simulink model "FullSystemSimGoed"  (R2020a)
settings: Solver=VariableStepAuto  StartTime=0.0  StopTime=T_sim  RelTol=1e-3
values from neighbouring files (symbols this model uses):
  a_friction = 0    [FullSystem.m]
  b_friction = 1.19    [FullSystem.m]
  C_T_matrix = ex2(2:12,2:12)'    [FullSystem.m]
  d_turbine = 0.15    [FullSystem.m]
  J_wind = 5.245e-6 * 1000    (= 0.005245)    [FullSystem.m]
  K_t = 0.023    [FullSystem.m]    (also in WindTurbine.m = 82.8991502528)
  K_v = 0.023 * pi / 30    (= 0.00240855436775)    [FullSystem.m]    (also in WindTurbine.m = 115.191730632)
  lambda_data_x = ex3(3, :)'    [FullSystem.m]
  lambda_opt = 2.8    [FullSystem.m]
  omega_0 = 1000    [FullSystem.m]    (also in SystemControl_script.m = 100:)
  P_max_EL = 3    [FullSystem.m]
  P_max_FC = 1    [FullSystem.m]
  P_max_LED = 12*0.16*4    (= 7.68)    [FullSystem.m]
  P_max_SP = 0.5    [FullSystem.m]
  P_max_WT = 0.2    [FullSystem.m]
  R_LED_max = 75/4    (= 18.75)    [FullSystem.m]
  r_LED_x = ex1(4, :)'    [FullSystem.m]
  r_PS_x = ex1(5,:)'    [FullSystem.m]
  r_SP_x = ex1(3, :)'    [FullSystem.m]
  r_wind_data_x = ex3(1, :)'    [FullSystem.m]
  r_WT_x = ex1(2, :)'    [FullSystem.m]
  rho_air = 1.225    [FullSystem.m]
  step_size = T_sim/n    (= 0.01)    [FullSystem.m]
  t_sample = pwm_timer/10    (= 0.01)    [FullSystem.m]
  T_sim = 10    [FullSystem.m]    (also in SystemControl_script.m; model_1.m = 24)
  V_w_data_x = ex3(2,:)'    [FullSystem.m]
undefined symbols (not defined in the file or in its folder): DiscIntNeverNeededParam
libraries: fl_lib x66, nesl_utility x55, ee_lib x12, eePwmGenerator x4, simulink x2
(part 1 of 2)
settings Model: Creator=thequ  LastModifiedBy=thequ
settings SolverCC: AlgebraicLoopSolver=LineSearch
settings DebuggingCC: ArithmeticOperatorsInVariantConditions=warning
settings SFSimCC: CustomCodeUndefinedFunction=UseInterfaceOnly

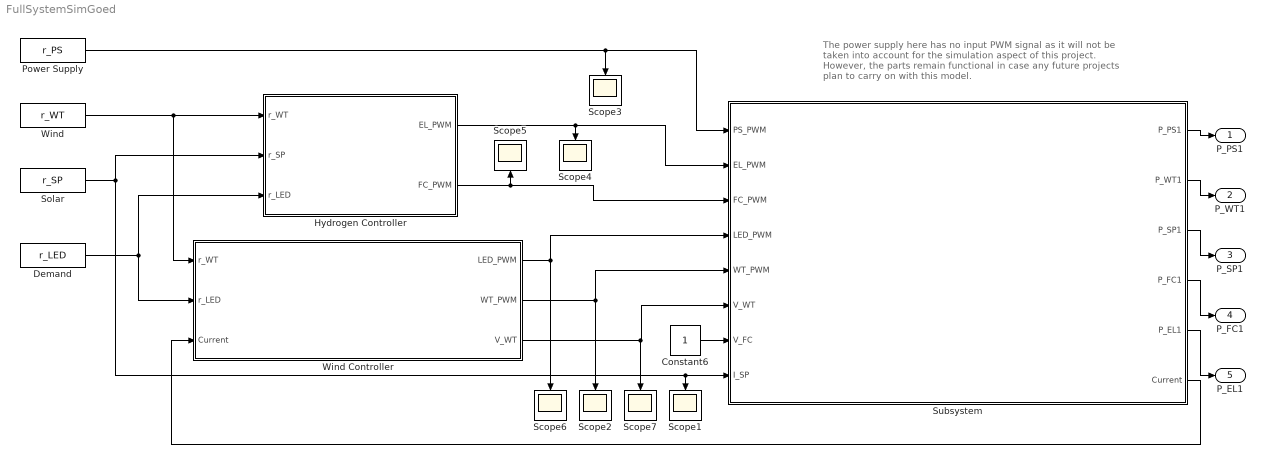
== system FullSystemSimGoed ==
  note: The power supply here has no input PWM signal as it will not
      | be taken into account for the simulation aspect of this project.
      | However, the parts remain functional in case any future
      | projects plan to carry on with this model.
  Constant6 : Constant
  Demand : FromWorkspace  VariableName=r_LED  SampleTime=T_sim/length(r_LED_x)  Interpolate=off  OutputAfterFinalValue=Holding final value
  Hydrogen Controller : Subsystem
  Power Supply : FromWorkspace  VariableName=r_PS  SampleTime=T_sim/length(r_PS_x)  Interpolate=off  OutputAfterFinalValue=Holding final value
  Scope{1..7} (7 alike) : Scope
  Solar : FromWorkspace  VariableName=r_SP  SampleTime=T_sim/length(r_SP_x)  Interpolate=off  OutputAfterFinalValue=Holding final value
  Subsystem : Subsystem
  Wind : FromWorkspace  VariableName=r_WT  SampleTime=T_sim/length(r_WT_x)  Interpolate=off  OutputAfterFinalValue=Holding final value
  Wind Controller : Subsystem
  P_PS1 : Outport
  P_WT1 : Outport  Port=2
  P_SP1 : Outport  Port=3
  P_FC1 : Outport  Port=4
  P_EL1 : Outport  Port=5
  wires:
  Subsystem/1(P_PS1) -> P_PS1/1
  Subsystem/2(P_WT1) -> P_WT1/1
  Subsystem/3(P_SP1) -> P_SP1/1
  Subsystem/4(P_FC1) -> P_FC1/1
  Subsystem/5(P_EL1) -> P_EL1/1
  Demand/1 -> Hydrogen Controller/3(r_LED), Wind Controller/2(r_LED)
  Constant6/1 -> Subsystem/7(V_FC)
  Wind/1 -> Wind Controller/1(r_WT), Hydrogen Controller/1(r_WT)
  Solar/1 -> Hydrogen Controller/2(r_SP), Subsystem/8(I_SP), Scope1/1
  Wind Controller/2(WT_PWM) -> Scope2/1, Subsystem/5(WT_PWM)
  Power Supply/1 -> Subsystem/1(PS_PWM), Scope3/1
  Hydrogen Controller/1(EL_PWM) -> Subsystem/2(EL_PWM), Scope4/1
  Hydrogen Controller/2(FC_PWM) -> Subsystem/3(FC_PWM), Scope5/1
  Wind Controller/1(LED_PWM) -> Scope6/1, Subsystem/4(LED_PWM)
  Wind Controller/3(V_WT) -> Scope7/1, Subsystem/6(V_WT)
  Subsystem/6(Current) -> Wind Controller/3(Current)

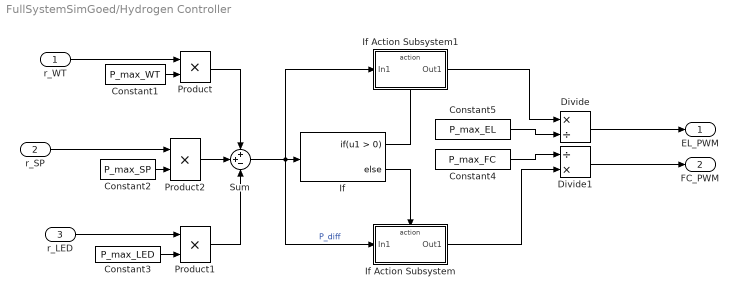
== system FullSystemSimGoed/Hydrogen Controller ==
  r_WT : Inport
  r_SP : Inport  Port=2
  r_LED : Inport  Port=3
  Constant1 : Constant  Value=P_max_WT
  Constant2 : Constant  Value=P_max_SP
  Constant3 : Constant  Value=P_max_LED
  Constant4 : Constant  Value=P_max_FC
  Constant5 : Constant  Value=P_max_EL
  Divide : Product  Inputs=*/
  Divide1 : Product  Inputs=/*
  If : If
  If Action Subsystem : Subsystem  TreatAsAtomicUnit=on
  If Action Subsystem1 : Subsystem  TreatAsAtomicUnit=on
  Product : Product
  Product1 : Product
  Product2 : Product
  Sum : Sum  Inputs=++-
  EL_PWM : Outport
  FC_PWM : Outport  Port=2
  wires:
  Divide1/1 -> FC_PWM/1
  Product/1 -> Sum/1
  Divide/1 -> EL_PWM/1
  r_WT/1 -> Product/1
  If Action Subsystem/1(Out1) -> Divide1/2
  Constant5/1 -> Divide/2
  If/2 -> If Action Subsystem/Action
  Product1/1 -> Sum/3
  Sum/1 -> If Action Subsystem1/1(In1), If Action Subsystem/1(In1), If/1  "P_diff"
  Constant1/1 -> Product/2
  Constant4/1 -> Divide1/1
  If/1 -> If Action Subsystem1/Action
  If Action Subsystem1/1(Out1) -> Divide/1
  Constant3/1 -> Product1/2
  Constant2/1 -> Product2/2
  Product2/1 -> Sum/2
  r_LED/1 -> Product1/1
  r_SP/1 -> Product2/1

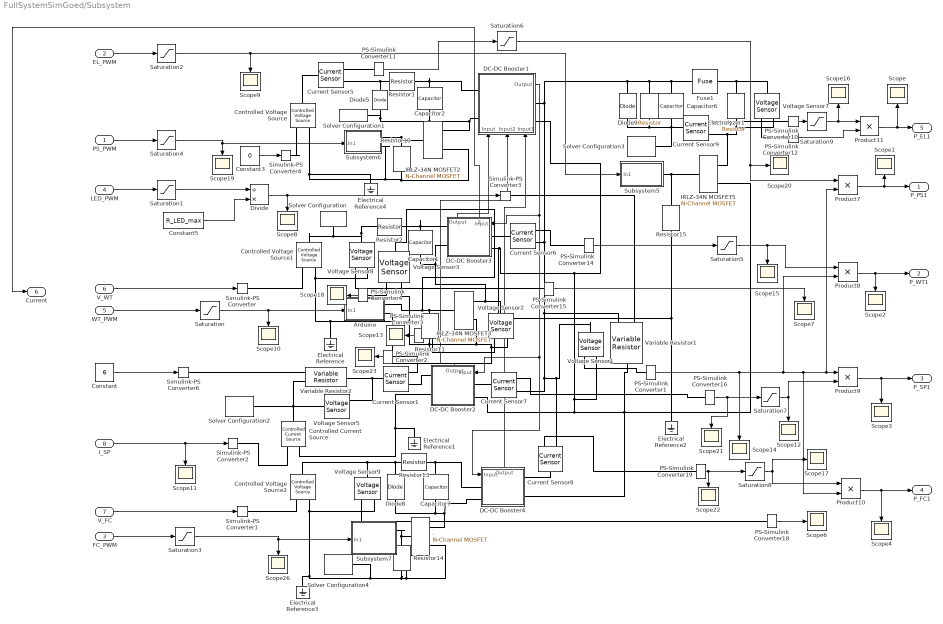
== system FullSystemSimGoed/Subsystem ==
  PS_PWM : Inport
  EL_PWM : Inport  Port=2
  FC_PWM : Inport  Port=3
  LED_PWM : Inport  Port=4
  WT_PWM : Inport  Port=5
  V_WT : Inport  Port=6
  V_FC : Inport  Port=7
  I_SP : Inport  Port=8
  " " : fl_lib/Electrical/Electrical Elements/Resistor  R=16 Ohm  i_specify=off  i_priority=None  i=0 A  i_nominal_specify=off  i_nominal_unit=A  i_nominal_value=1  v_specify=off  v_priority=None  v=0 V  v_nominal_specify=off  v_nominal_unit=V  v_nominal_value=1
  . : ee_lib/Semiconductors & Converters/N-Channel MOSFET  paramTerminal=ee.enum.mosfet.numberOfTerminals.three  parameterization=1  prmDatasheet=1  prmEquCoeff=1  Beta=5.0 A/V^2  Rds=0.046 Ohm  Id=30 A  Vgs=5 V  Vth=1.5 V  Vth0=1.7 V  lam=0 1/V  gamma_vth=0.5 V^0.50000  phib=0.5 V  Vth1=1.9071 V  Vbs1=-1 V  Vth2=2.066 V  Vbs2=-2 V  Tmeas=25 degC  RS=0.0001 Ohm  RD=0.01 Ohm  RB=0.001 Ohm  C_param=1  C_GS=270 pF  C_GD=80 pF  C_DS=0 pF  C_iss=350 pF  C_rss=80 pF  C_oss=0 pF  charge_linearity_param=1  C_OX=200 pF  V_C_OX=-0.5 V  C_iss_vec=[720, 700, 590, 470, 390, 310] pF  C_rss_vec=[450, 400, 300, 190, 95, 55] pF  C_oss_vec=[900, 810, 690, 420, 270, 170] pF  C_GS_vec=[270, 300, 290, 280, 295, 255] pF  C_GD_vec=[450, 400, 300, 190, 95, 55] pF  C_DS_vec=[450, 410, 390, 230, 175, 115] pF  C_Vds_vec=[.1, .3, 1, 3, 10, 30] V  V_GS_for_cap_data=0 V  charge_linearity_param_vgb=ee.enum.mosfet.cgbLinearity.instantly  IsDiode=0 A  Vbi=0.6 V  n=1  Cj0Diode=0 pF  TT=50e-9 s  dVth_dT=-6 mV/K  dVth0_dT=-6 mV/K  Rds_T2=0.037 Ohm  Tmeas2=125 degC  BEXDatasheet=-1.5  BEXEquCoeff=-1.5  etaisDatasheet=3  etaisEquCoeff=3  TdeviceDatasheet=25 degC  TdeviceEquCoeff=25 degC  thermal_network_parameterization=ee.enum.thermalNetworkTopology.cauer  Rth=[0, 10] K/W  Rth_Foster=[4, 6] K/W  thermal_mass_parameterization=ee.enum.thermalNetwork.timeconstant  thermal_mass=[0, 1] J/K  thermal_mass_Foster=[1.5, 3] J/K  thermal_time_constant=[0, 10] s  thermal_time_constant_Foster=[6, 18] s  thermal_mass_initial_temperatures=[25, 25] degC  betaref=18 A/V^2  Vfbref=-1.1 V  gamma=3.5 V^0.50000  phib2ref=1 V  thesatref=0.4 1/V  alpha=0  Vp=5e-2 V  thesrref=0 1/V  m=8  Tref=25 degC  Cox=1500 pF  Cgso=100 pF  Cgdo=14 pF  Rsref=2e-3 Ohm  Rdref=0.17 Ohm  Rgref=8.4 Ohm  Rbref=2e-3 Ohm  Isref=5.2e-13 A  Cj0=480 pF  Tprm=1  etabet=1.3  Stvfb=5e-4 V/K  Stphib=-8.5e-4 V/K  etasat=1.04  etasr=0.65  etar=0.95  etais=3  Tsim=25 degC  T0=[25, 25] degC
  Arduino : Subsystem
  Capacitor1 : fl_lib/Electrical/Electrical Elements/Capacitor  c=1000 uF  r=0.02 Ohm  g=0 1/Ohm  i_specify=off  i_priority=None  i=0 A  i_nominal_specify=off  i_nominal_unit=A  i_nominal_value=1  v_specify=off  v_priority=None  v=0 V  v_nominal_specify=off  v_nominal_unit=V  v_nominal_value=1  vc_specify=off  vc_priority=High  vc=0 V  vc_nominal_specify=off  vc_nominal_unit=V  vc_nominal_value=1
  Capacitor2 : fl_lib/Electrical/Electrical Elements/Capacitor  c=1000 uF  r=0.02 Ohm  g=0 1/Ohm  i_specify=off  i_priority=None  i=0 A  i_nominal_specify=off  i_nominal_unit=A  i_nominal_value=1  v_specify=off  v_priority=None  v=0 V  v_nominal_specify=off  v_nominal_unit=V  v_nominal_value=1  vc_specify=off  vc_priority=High  vc=0 V  vc_nominal_specify=off  vc_nominal_unit=V  vc_nominal_value=1
  Capacitor6 : fl_lib/Electrical/Electrical Elements/Capacitor  c=1000 uF  r=0.20 Ohm  g=0 1/Ohm  i_specify=off  i_priority=None  i=0 A  i_nominal_specify=off  i_nominal_unit=A  i_nominal_value=1  v_specify=off  v_priority=None  v=0 V  v_nominal_specify=off  v_nominal_unit=V  v_nominal_value=1  vc_specify=off  vc_priority=High  vc=0 V  vc_nominal_specify=off  vc_nominal_unit=V  vc_nominal_value=1
  Capacitor7 : fl_lib/Electrical/Electrical Elements/Capacitor  c=1000 uF  r=0.02 Ohm  g=0 1/Ohm  i_specify=off  i_priority=None  i=0 A  i_nominal_specify=off  i_nominal_unit=A  i_nominal_value=1  v_specify=off  v_priority=None  v=0 V  v_nominal_specify=off  v_nominal_unit=V  v_nominal_value=1  vc_specify=off  vc_priority=High  vc=0 V  vc_nominal_specify=off  vc_nominal_unit=V  vc_nominal_value=1
  Constant : Constant  Value=6
  Constant3 : Constant  Value=0
  Constant5 : Constant  Value=R_LED_max
  Controlled Current Source : fl_lib/Electrical/Electrical Sources/Controlled Current Source
  Controlled Voltage Source : fl_lib/Electrical/Electrical Sources/Controlled Voltage Source
  Controlled Voltage Source1 : fl_lib/Electrical/Electrical Sources/Controlled Voltage Source
  Controlled Voltage Source2 : fl_lib/Electrical/Electrical Sources/Controlled Voltage Source
  Current Sensor{1,5..9} (6 alike) : fl_lib/Electrical/Electrical Sensors/Current Sensor
  DC-DC Booster1 : Subsystem
      settings: PortSchema="{\"entries\":[{\"content\":{\"sides\":[{\"content\":{\"connectorIds\":[\"LConn1\",\"LConn2\"]},\"type\":\"ConnectorPlacement.EquallySpacedRectSide\",\"uuid\":\"3f87025d-e72c-4f7c-9c78-5492fcc5bb7b\"},{\"content\":{\"connectorIds\":[\"Out1\",\"RConn1\",\"RConn2\"],\"side\":\"RIGHT\"},\"type\":\"ConnectorPlacement.EquallySpacedRectSide\",\"uuid\":\"8496db32-d1b8-4ca7-babe-2510a055e486\"},{\"content\":{\"connectorIds\":[],\"side\":\"TOP\"},\"type\":\"ConnectorPlacement.EquallySpacedRectSide\",\"uuid\":\"d85b2c98-f560-4129-a6ac-6fa684551bcf\"},{\"content\":{\"connectorIds\":[\"In1\",\"In2\",\"In3\"],\"side\":\"BOTTOM\"},\"type\":\"ConnectorPlacement.EquallySpacedRectSide\",\"uuid\":\"fe0eaf9c-8c75-4de4-84e6-0314a1617f55\"}]},\"type\":\"ConnectorPlacement.EquallySpacedConnector\",\"uuid\":\"a6ed506c-6875-4055-9614-7dad2b572790\"}],\"packageUris\":[\"http://schema.mathworks.com/mf0/Connector/19700101\"],\"version\":\"1.0\"}"
  DC-DC Booster2 : Subsystem
      settings: PortSchema="{\"entries\":[{\"content\":{\"sides\":[{\"content\":{\"connectorIds\":[\"LConn1\",\"LConn2\"]},\"type\":\"ConnectorPlacement.EquallySpacedRectSide\",\"uuid\":\"e779e15f-05fe-47ae-aa08-5379ba170b98\"},{\"content\":{\"connectorIds\":[\"In1\",\"RConn1\",\"RConn2\"],\"side\":\"RIGHT\"},\"type\":\"ConnectorPlacement.EquallySpacedRectSide\",\"uuid\":\"c806a98b-8847-4c98-ba30-df3a6a47e20e\"},{\"content\":{\"connectorIds\":[\"Out1\"],\"side\":\"TOP\"},\"type\":\"ConnectorPlacement.EquallySpacedRectSide\",\"uuid\":\"f525c8fa-41c3-4ddc-a882-4dcfcc470e8d\"}]},\"type\":\"ConnectorPlacement.EquallySpacedConnector\",\"uuid\":\"8e1dab04-976c-405f-8e86-df668b770438\"}],\"packageUris\":[\"http://schema.mathworks.com/mf0/Connector/19700101\"],\"version\":\"1.0\"}"
  DC-DC Booster3 : Subsystem
      settings: PortSchema="{\"entries\":[{\"content\":{\"sides\":[{\"content\":{\"connectorIds\":[\"LConn1\",\"LConn2\"]},\"type\":\"ConnectorPlacement.EquallySpacedRectSide\",\"uuid\":\"e779e15f-05fe-47ae-aa08-5379ba170b98\"},{\"content\":{\"connectorIds\":[\"In1\",\"RConn1\",\"RConn2\"],\"side\":\"RIGHT\"},\"type\":\"ConnectorPlacement.EquallySpacedRectSide\",\"uuid\":\"c806a98b-8847-4c98-ba30-df3a6a47e20e\"},{\"content\":{\"connectorIds\":[\"Out1\",\"Out2\"],\"side\":\"TOP\"},\"type\":\"ConnectorPlacement.EquallySpacedRectSide\",\"uuid\":\"f525c8fa-41c3-4ddc-a882-4dcfcc470e8d\"}]},\"type\":\"ConnectorPlacement.EquallySpacedConnector\",\"uuid\":\"8e1dab04-976c-405f-8e86-df668b770438\"}],\"packageUris\":[\"http://schema.mathworks.com/mf0/Connector/19700101\"],\"version\":\"1.0\"}"
  DC-DC Booster4 : Subsystem
      settings: PortSchema="{\"entries\":[{\"content\":{\"sides\":[{\"content\":{\"connectorIds\":[\"In1\",\"LConn1\",\"LConn2\"]},\"type\":\"ConnectorPlacement.EquallySpacedRectSide\",\"uuid\":\"53e27ef1-b6e4-4838-a313-2833a9f48f28\"},{\"content\":{\"connectorIds\":[\"RConn1\",\"RConn2\"],\"side\":\"RIGHT\"},\"type\":\"ConnectorPlacement.EquallySpacedRectSide\",\"uuid\":\"d6eb4206-926e-4a9e-8f3b-898e00b2f09a\"},{\"content\":{\"connectorIds\":[\"Out1\"],\"side\":\"TOP\"},\"type\":\"ConnectorPlacement.EquallySpacedRectSide\",\"uuid\":\"2a6192b7-9850-4397-b133-a2a3e44eb736\"}]},\"type\":\"ConnectorPlacement.EquallySpacedConnector\",\"uuid\":\"90d1bf23-e581-4b0f-8608-623e9f776cda\"}],\"packageUris\":[\"http://schema.mathworks.com/mf0/Connector/19700101\"],\"version\":\"1.0\"}"
  Diode5 : ee_lib/Semiconductors & Converters/Diode  ModelType=ee.enum.diode.modelType.pwl  Vf=0.6 V  Ron=0.3 Ohm  Goff=1e-8 S  prmExp=ee.enum.diode.expParam.useTwo  I12=[.0137, .545] A  V12=[.6, .7] V  IS=1e-12 A  ec=1  I1=0.0137 A  V1=0.6 V  RS=0 Ohm  Tmeas=25 degC  N_series=1  N_parallel=1  Rz=0.3 Ohm  BV=inf V  C_param=ee.enum.diode.capParam.fixed  CJ=5 pF  CJ0=5 pF  VJ=1 V  Mgrad=0.5  Vvec=[.1, 10, 100] V  Cvec=[3.5, 1, .4] pF  FC=0.5  Q_param=ee.enum.diode.recoveryParam.off  iRM=-7.15 A  iF=4 A  didt=-750 A/us  trr_factor=3  trr=115 ns  Qrr=1500 s*uA  TT=50 ns  tau=100 ns  T_param=ee.enum.diode.temperatureParam.off  IS_T2=1.25e-7 A  I1_T2=0.245 A  V1_T2=0.5 V  Tmeas2=125 degC  EG_param=ee.enum.diode.egapParam.material_si  EG=1.11 eV  XTI_param=ee.enum.diode.xtiParam.pn  XTI=3  dBVdT=0 V/K  Tdevice=25 degC  i_specify=off  i_priority=None  i=0 A  i_nominal_specify=off  i_nominal_unit=A  i_nominal_value=1  v_specify=off  v_priority=None  v=0 V  v_nominal_specify=off  v_nominal_unit=V  v_nominal_value=1  i_capacitor_specify=off  i_capacitor_priority=None  i_capacitor=0 A  i_capacitor_nominal_specify=off  i_capacitor_nominal_unit=A  i_capacitor_nominal_value=1  v_capacitor_specify=off  v_capacitor_priority=None  v_capacitor=0 V  v_capacitor_nominal_specify=off  v_capacitor_nominal_unit=V  v_capacitor_nominal_value=1  power_dissipated_specify=off  power_dissipated_priority=None  power_dissipated=0 W  power_dissipated_nominal_specify=off  power_dissipated_nominal_unit=W  power_dissipated_nominal_value=1  thermal_network_parameterization=ee.enum.thermalNetworkTopology.cauer  Rth=[0, 10] K/W  Rth_Foster=[4, 6] K/W  thermal_mass_parameterization=ee.enum.thermalNetwork.timeconstant  thermal_mass=[0, 1] J/K  thermal_mass_Foster=[1.5, 3] J/K  thermal_time_constant=[0, 10] s  thermal_time_constant_Foster=[6, 18] s  thermal_mass_initial_temperatures=[25, 25] degC
  Diode8 : ee_lib/Semiconductors & Converters/Diode  ModelType=ee.enum.diode.modelType.pwl  Vf=0.85 V  Ron=0.05 Ohm  Goff=1e-8 S  prmExp=ee.enum.diode.expParam.useTwo  I12=[.0137, .545] A  V12=[.6, .7] V  IS=1e-12 A  ec=1  I1=0.0137 A  V1=0.6 V  RS=0 Ohm  Tmeas=25 degC  N_series=1  N_parallel=1  Rz=0.3 Ohm  BV=inf V  C_param=ee.enum.diode.capParam.fixed  CJ=5 pF  CJ0=5 pF  VJ=1 V  Mgrad=0.5  Vvec=[.1, 10, 100] V  Cvec=[3.5, 1, .4] pF  FC=0.5  Q_param=ee.enum.diode.recoveryParam.off  iRM=-7.15 A  iF=4 A  didt=-750 A/us  trr_factor=3  trr=115 ns  Qrr=1500 s*uA  TT=50 ns  tau=100 ns  T_param=ee.enum.diode.temperatureParam.off  IS_T2=1.25e-7 A  I1_T2=0.245 A  V1_T2=0.5 V  Tmeas2=125 degC  EG_param=ee.enum.diode.egapParam.material_si  EG=1.11 eV  XTI_param=ee.enum.diode.xtiParam.pn  XTI=3  dBVdT=0 V/K  Tdevice=25 degC  i_specify=off  i_priority=None  i=0 A  i_nominal_specify=off  i_nominal_unit=A  i_nominal_value=1  v_specify=off  v_priority=None  v=0 V  v_nominal_specify=off  v_nominal_unit=V  v_nominal_value=1  i_capacitor_specify=off  i_capacitor_priority=None  i_capacitor=0 A  i_capacitor_nominal_specify=off  i_capacitor_nominal_unit=A  i_capacitor_nominal_value=1  v_capacitor_specify=off  v_capacitor_priority=None  v_capacitor=0 V  v_capacitor_nominal_specify=off  v_capacitor_nominal_unit=V  v_capacitor_nominal_value=1  power_dissipated_specify=off  power_dissipated_priority=None  power_dissipated=0 W  power_dissipated_nominal_specify=off  power_dissipated_nominal_unit=W  power_dissipated_nominal_value=1  thermal_network_parameterization=ee.enum.thermalNetworkTopology.cauer  Rth=[0, 10] K/W  Rth_Foster=[4, 6] K/W  thermal_mass_parameterization=ee.enum.thermalNetwork.timeconstant  thermal_mass=[0, 1] J/K  thermal_mass_Foster=[1.5, 3] J/K  thermal_time_constant=[0, 10] s  thermal_time_constant_Foster=[6, 18] s  thermal_mass_initial_temperatures=[25, 25] degC
  Diode9 : ee_lib/Semiconductors & Converters/Diode  ModelType=ee.enum.diode.modelType.pwl  Vf=0.7 V  Ron=0.3 Ohm  Goff=1e-8 S  prmExp=ee.enum.diode.expParam.useTwo  I12=[.0137, .545] A  V12=[.6, .7] V  IS=1e-12 A  ec=1  I1=0.0137 A  V1=0.6 V  RS=0 Ohm  Tmeas=25 degC  N_series=1  N_parallel=1  Rz=0.3 Ohm  BV=inf V  C_param=ee.enum.diode.capParam.fixed  CJ=5 pF  CJ0=5 pF  VJ=1 V  Mgrad=0.5  Vvec=[.1, 10, 100] V  Cvec=[3.5, 1, .4] pF  FC=0.5  Q_param=ee.enum.diode.recoveryParam.off  iRM=-7.15 A  iF=4 A  didt=-750 A/us  trr_factor=3  trr=115 ns  Qrr=1500 s*uA  TT=50 ns  tau=100 ns  T_param=ee.enum.diode.temperatureParam.off  IS_T2=1.25e-7 A  I1_T2=0.245 A  V1_T2=0.5 V  Tmeas2=125 degC  EG_param=ee.enum.diode.egapParam.material_si  EG=1.11 eV  XTI_param=ee.enum.diode.xtiParam.pn  XTI=3  dBVdT=0 V/K  Tdevice=25 degC  i_specify=off  i_priority=None  i=0 A  i_nominal_specify=off  i_nominal_unit=A  i_nominal_value=1  v_specify=off  v_priority=None  v=0 V  v_nominal_specify=off  v_nominal_unit=V  v_nominal_value=1  i_capacitor_specify=off  i_capacitor_priority=None  i_capacitor=0 A  i_capacitor_nominal_specify=off  i_capacitor_nominal_unit=A  i_capacitor_nominal_value=1  v_capacitor_specify=off  v_capacitor_priority=None  v_capacitor=0 V  v_capacitor_nominal_specify=off  v_capacitor_nominal_unit=V  v_capacitor_nominal_value=1  power_dissipated_specify=off  power_dissipated_priority=None  power_dissipated=0 W  power_dissipated_nominal_specify=off  power_dissipated_nominal_unit=W  power_dissipated_nominal_value=1  thermal_network_parameterization=ee.enum.thermalNetworkTopology.cauer  Rth=[0, 10] K/W  Rth_Foster=[4, 6] K/W  thermal_mass_parameterization=ee.enum.thermalNetwork.timeconstant  thermal_mass=[0, 1] J/K  thermal_mass_Foster=[1.5, 3] J/K  thermal_time_constant=[0, 10] s  thermal_time_constant_Foster=[6, 18] s  thermal_mass_initial_temperatures=[25, 25] degC
  Divide : Product  Inputs=/*
  Electrical Reference{,1..4} (5 alike) : fl_lib/Electrical/Electrical Elements/Electrical Reference
  Electrolyzer1 : fl_lib/Electrical/Electrical Elements/Resistor  R=4 Ohm  i_specify=off  i_priority=None  i=0 A  i_nominal_specify=off  i_nominal_unit=A  i_nominal_value=1  v_specify=off  v_priority=None  v=0 V  v_nominal_specify=off  v_nominal_unit=V  v_nominal_value=1
  Fuse1 : ee_lib/Switches & Breakers/Fuse  prm=1  I_rated=1.5 A  melt_margin=1  T_fuse=0 s  I2t=1 s*A^2  I_vec=[1.9, 2, 2.5, 30] A  t_vec=[10000, 1, .3, .001] s  R_closed=0.01 Ohm  G_open=1e-8 1/Ohm  exposemeasurement=ee.enum.exposemeasurement.hidden
      settings: SourceProductBaseCode=PS  InternalSimscapePortConfiguration="{\"Bottom\":[],\"Left\":[{\"id\":\"p\",\"label\":\"\",\"type\":\"foundation.electrical.electrical\"}],\"Right\":[{\"id\":\"n\",\"label\":\"\",\"type\":\"foundation.electrical.electrical\"}],\"Top\":[]}"
  IRLZ-34N MOSFET2 : ee_lib/Semiconductors & Converters/N-Channel MOSFET  paramTerminal=ee.enum.mosfet.numberOfTerminals.three  parameterization=1  prmDatasheet=1  prmEquCoeff=1  Beta=5.0 A/V^2  Rds=0.046 Ohm  Id=30 A  Vgs=5 V  Vth=1.5 V  Vth0=1.7 V  lam=0 1/V  gamma_vth=0.5 V^0.50000  phib=0.5 V  Vth1=1.9071 V  Vbs1=-1 V  Vth2=2.066 V  Vbs2=-2 V  Tmeas=25 degC  RS=0.0001 Ohm  RD=0.01 Ohm  RB=0.001 Ohm  C_param=1  C_GS=270 pF  C_GD=80 pF  C_DS=0 pF  C_iss=350 pF  C_rss=80 pF  C_oss=0 pF  charge_linearity_param=1  C_OX=200 pF  V_C_OX=-0.5 V  C_iss_vec=[720, 700, 590, 470, 390, 310] pF  C_rss_vec=[450, 400, 300, 190, 95, 55] pF  C_oss_vec=[900, 810, 690, 420, 270, 170] pF  C_GS_vec=[270, 300, 290, 280, 295, 255] pF  C_GD_vec=[450, 400, 300, 190, 95, 55] pF  C_DS_vec=[450, 410, 390, 230, 175, 115] pF  C_Vds_vec=[.1, .3, 1, 3, 10, 30] V  V_GS_for_cap_data=0 V  charge_linearity_param_vgb=ee.enum.mosfet.cgbLinearity.instantly  IsDiode=0 A  Vbi=0.6 V  n=1  Cj0Diode=0 pF  TT=50e-9 s  dVth_dT=-6 mV/K  dVth0_dT=-6 mV/K  Rds_T2=0.037 Ohm  Tmeas2=125 degC  BEXDatasheet=-1.5  BEXEquCoeff=-1.5  etaisDatasheet=3  etaisEquCoeff=3  TdeviceDatasheet=25 degC  TdeviceEquCoeff=25 degC  thermal_network_parameterization=ee.enum.thermalNetworkTopology.cauer  Rth=[0, 10] K/W  Rth_Foster=[4, 6] K/W  thermal_mass_parameterization=ee.enum.thermalNetwork.timeconstant  thermal_mass=[0, 1] J/K  thermal_mass_Foster=[1.5, 3] J/K  thermal_time_constant=[0, 10] s  thermal_time_constant_Foster=[6, 18] s  thermal_mass_initial_temperatures=[25, 25] degC  betaref=18 A/V^2  Vfbref=-1.1 V  gamma=3.5 V^0.50000  phib2ref=1 V  thesatref=0.4 1/V  alpha=0  Vp=5e-2 V  thesrref=0 1/V  m=8  Tref=25 degC  Cox=1500 pF  Cgso=100 pF  Cgdo=14 pF  Rsref=2e-3 Ohm  Rdref=0.17 Ohm  Rgref=8.4 Ohm  Rbref=2e-3 Ohm  Isref=5.2e-13 A  Cj0=480 pF  Tprm=1  etabet=1.3  Stvfb=5e-4 V/K  Stphib=-8.5e-4 V/K  etasat=1.04  etasr=0.65  etar=0.95  etais=3  Tsim=25 degC  T0=[25, 25] degC
  IRLZ-34N MOSFET3 : ee_lib/Semiconductors & Converters/N-Channel MOSFET  paramTerminal=ee.enum.mosfet.numberOfTerminals.three  parameterization=1  prmDatasheet=1  prmEquCoeff=1  Beta=5.0 A/V^2  Rds=0.046 Ohm  Id=30 A  Vgs=5 V  Vth=1.5 V  Vth0=1.7 V  lam=0 1/V  gamma_vth=0.5 V^0.50000  phib=0.5 V  Vth1=1.9071 V  Vbs1=-1 V  Vth2=2.066 V  Vbs2=-2 V  Tmeas=25 degC  RS=0.0001 Ohm  RD=0.01 Ohm  RB=0.001 Ohm  C_param=1  C_GS=270 pF  C_GD=80 pF  C_DS=0 pF  C_iss=350 pF  C_rss=80 pF  C_oss=0 pF  charge_linearity_param=1  C_OX=200 pF  V_C_OX=-0.5 V  C_iss_vec=[720, 700, 590, 470, 390, 310] pF  C_rss_vec=[450, 400, 300, 190, 95, 55] pF  C_oss_vec=[900, 810, 690, 420, 270, 170] pF  C_GS_vec=[270, 300, 290, 280, 295, 255] pF  C_GD_vec=[450, 400, 300, 190, 95, 55] pF  C_DS_vec=[450, 410, 390, 230, 175, 115] pF  C_Vds_vec=[.1, .3, 1, 3, 10, 30] V  V_GS_for_cap_data=0 V  charge_linearity_param_vgb=ee.enum.mosfet.cgbLinearity.instantly  IsDiode=0 A  Vbi=0.6 V  n=1  Cj0Diode=0 pF  TT=50e-9 s  dVth_dT=-6 mV/K  dVth0_dT=-6 mV/K  Rds_T2=0.037 Ohm  Tmeas2=125 degC  BEXDatasheet=-1.5  BEXEquCoeff=-1.5  etaisDatasheet=3  etaisEquCoeff=3  TdeviceDatasheet=25 degC  TdeviceEquCoeff=25 degC  thermal_network_parameterization=ee.enum.thermalNetworkTopology.cauer  Rth=[0, 10] K/W  Rth_Foster=[4, 6] K/W  thermal_mass_parameterization=ee.enum.thermalNetwork.timeconstant  thermal_mass=[0, 1] J/K  thermal_mass_Foster=[1.5, 3] J/K  thermal_time_constant=[0, 10] s  thermal_time_constant_Foster=[6, 18] s  thermal_mass_initial_temperatures=[25, 25] degC  betaref=18 A/V^2  Vfbref=-1.1 V  gamma=3.5 V^0.50000  phib2ref=1 V  thesatref=0.4 1/V  alpha=0  Vp=5e-2 V  thesrref=0 1/V  m=8  Tref=25 degC  Cox=1500 pF  Cgso=100 pF  Cgdo=14 pF  Rsref=2e-3 Ohm  Rdref=0.17 Ohm  Rgref=8.4 Ohm  Rbref=2e-3 Ohm  Isref=5.2e-13 A  Cj0=480 pF  Tprm=1  etabet=1.3  Stvfb=5e-4 V/K  Stphib=-8.5e-4 V/K  etasat=1.04  etasr=0.65  etar=0.95  etais=3  Tsim=25 degC  T0=[25, 25] degC
  IRLZ-34N MOSFET5 : ee_lib/Semiconductors & Converters/N-Channel MOSFET  paramTerminal=ee.enum.mosfet.numberOfTerminals.three  parameterization=1  prmDatasheet=1  prmEquCoeff=1  Beta=5.0 A/V^2  Rds=0.046 Ohm  Id=30 A  Vgs=5 V  Vth=1.5 V  Vth0=1.7 V  lam=0 1/V  gamma_vth=0.5 V^0.50000  phib=0.5 V  Vth1=1.9071 V  Vbs1=-1 V  Vth2=2.066 V  Vbs2=-2 V  Tmeas=25 degC  RS=0.0001 Ohm  RD=0.01 Ohm  RB=0.001 Ohm  C_param=1  C_GS=270 pF  C_GD=80 pF  C_DS=0 pF  C_iss=350 pF  C_rss=80 pF  C_oss=0 pF  charge_linearity_param=1  C_OX=200 pF  V_C_OX=-0.5 V  C_iss_vec=[720, 700, 590, 470, 390, 310] pF  C_rss_vec=[450, 400, 300, 190, 95, 55] pF  C_oss_vec=[900, 810, 690, 420, 270, 170] pF  C_GS_vec=[270, 300, 290, 280, 295, 255] pF  C_GD_vec=[450, 400, 300, 190, 95, 55] pF  C_DS_vec=[450, 410, 390, 230, 175, 115] pF  C_Vds_vec=[.1, .3, 1, 3, 10, 30] V  V_GS_for_cap_data=0 V  charge_linearity_param_vgb=ee.enum.mosfet.cgbLinearity.instantly  IsDiode=0 A  Vbi=0.6 V  n=1  Cj0Diode=0 pF  TT=50e-9 s  dVth_dT=-6 mV/K  dVth0_dT=-6 mV/K  Rds_T2=0.037 Ohm  Tmeas2=125 degC  BEXDatasheet=-1.5  BEXEquCoeff=-1.5  etaisDatasheet=3  etaisEquCoeff=3  TdeviceDatasheet=25 degC  TdeviceEquCoeff=25 degC  thermal_network_parameterization=ee.enum.thermalNetworkTopology.cauer  Rth=[0, 10] K/W  Rth_Foster=[4, 6] K/W  thermal_mass_parameterization=ee.enum.thermalNetwork.timeconstant  thermal_mass=[0, 1] J/K  thermal_mass_Foster=[1.5, 3] J/K  thermal_time_constant=[0, 10] s  thermal_time_constant_Foster=[6, 18] s  thermal_mass_initial_temperatures=[25, 25] degC  betaref=18 A/V^2  Vfbref=-1.1 V  gamma=3.5 V^0.50000  phib2ref=1 V  thesatref=0.4 1/V  alpha=0  Vp=5e-2 V  thesrref=0 1/V  m=8  Tref=25 degC  Cox=1500 pF  Cgso=100 pF  Cgdo=14 pF  Rsref=2e-3 Ohm  Rdref=0.17 Ohm  Rgref=8.4 Ohm  Rbref=2e-3 Ohm  Isref=5.2e-13 A  Cj0=480 pF  Tprm=1  etabet=1.3  Stvfb=5e-4 V/K  Stphib=-8.5e-4 V/K  etasat=1.04  etasr=0.65  etar=0.95  etais=3  Tsim=25 degC  T0=[25, 25] degC
  PS-Simulink Converter{1..4,10..12,14..16,18..19} (12 alike) : nesl_utility/PS-Simulink Converter  PhysicalDomain=network_engine_domain  SubClassName=ps_output  LeftPortType=input  RightPortType=output  PseudoPeriodic=off  Frequencies=[]  Unit=inherit  AffineConversion=off
  Product{7..11} (5 alike) : Product
  Resistor1 : fl_lib/Electrical/Electrical Elements/Resistor  R=16 Ohm  i_specify=off  i_priority=None  i=0 A  i_nominal_specify=off  i_nominal_unit=A  i_nominal_value=1  v_specify=off  v_priority=None  v=0 V  v_nominal_specify=off  v_nominal_unit=V  v_nominal_value=1
  Resistor{10..11,14..15} (4 alike) : fl_lib/Electrical/Electrical Elements/Resistor  R=10000 Ohm  i_specify=off  i_priority=None  i=0 A  i_nominal_specify=off  i_nominal_unit=A  i_nominal_value=1  v_specify=off  v_priority=None  v=0 V  v_nominal_specify=off  v_nominal_unit=V  v_nominal_value=1
  Resistor13 : fl_lib/Electrical/Electrical Elements/Resistor  R=16 Ohm  i_specify=off  i_priority=None  i=0 A  i_nominal_specify=off  i_nominal_unit=A  i_nominal_value=1  v_specify=off  v_priority=None  v=0 V  v_nominal_specify=off  v_nominal_unit=V  v_nominal_value=1
  Resistor2 : fl_lib/Electrical/Electrical Elements/Resistor  R=16 Ohm  i_specify=off  i_priority=None  i=0 A  i_nominal_specify=off  i_nominal_unit=A  i_nominal_value=1  v_specify=off  v_priority=None  v=0 V  v_nominal_specify=off  v_nominal_unit=V  v_nominal_value=1
  Saturation{,1..4,7} (6 alike) : Saturate  UpperLimit=1  LowerLimit=0
  Saturation5 : Saturate  UpperLimit=2
  Saturation6 : Saturate  UpperLimit=2
  Saturation8 : Saturate
  Saturation9 : Saturate  UpperLimit=2  LowerLimit=0
  Scope{,1..4,6..23,26} (24 alike) : Scope
  Simulink-PS Converter : nesl_utility/Simulink-PS Converter  PhysicalDomain=network_engine_domain  SubClassName=ps_input  LeftPortType=input  RightPortType=output  PseudoPeriodic=off  Frequencies=[]  NoiseDistribution=none  NoiseParameters=[]  Unit=1  AffineConversion=off  FilteringAndDerivatives=filter  SimscapeFilterOrder=1  InputFilterTimeConstant=0.001  UdotUserProvided=0
  Simulink-PS Converter{1,3..4,6} (4 alike) : nesl_utility/Simulink-PS Converter  PhysicalDomain=network_engine_domain  SubClassName=ps_input  LeftPortType=input  RightPortType=output  PseudoPeriodic=off  Frequencies=[]  NoiseDistribution=none  NoiseParameters=[]  Unit=1  AffineConversion=off  FilteringAndDerivatives=provide  SimscapeFilterOrder=1  InputFilterTimeConstant=0.001  UdotUserProvided=0
  Simulink-PS Converter2 : nesl_utility/Simulink-PS Converter  PhysicalDomain=network_engine_domain  SubClassName=ps_input  LeftPortType=input  RightPortType=output  PseudoPeriodic=off  Frequencies=[]  NoiseDistribution=none  NoiseParameters=[]  Unit=1  AffineConversion=off  FilteringAndDerivatives=filter  SimscapeFilterOrder=1  InputFilterTimeConstant=0.001  UdotUserProvided=0
  Solver Configuration{,1..4} (5 alike) : nesl_utility/Solver Configuration  PhysicalDomain=network_engine_domain  SubClassName=solver  LeftPortType=input  RightPortType=generic  Tones=[]  Harmonics=[]  SimulateNoise=off  Profile=off  UseLocalSampling=off  EnableSwitchedLinearOptims=on  FrequencyDomain=off  UseCCode=off  RelTol=0.001  AbsTol=1e-06  MinStep=1e-09  ToWorkspace=off  RevertToSquareIcSolve=off  NumHomotopyIterations=100  PhasorMode=off  PhasorModeNumHarmonics=1  DoDC=off  ResidualTolerance=1e-09  UseLocalSolver=off  LocalSolverChoice=NE_BACKWARD_EULER_ADVANCER  LocalSolverSampleTime=0.001  DoFixedCost=off  MaxNonlinIter=3  MaxModeIter=2  LinearAlgebra=auto  EquationFormulation=NE_TIME_EF  DelaysMemoryBudget=1024  AutomaticFiltering=on  FilteringTimeConstant=0.001  PartitionStorageMethod=AS_NEEDED  PartitionMemoryBudget=1024  PartitionMethod=ROBUST
  Subsystem5 : Subsystem
  Subsystem6 : Subsystem
  Subsystem7 : Subsystem
  Variable Resistor1 : fl_lib/Electrical/Electrical Elements/Variable Resistor  Rmin=1 Ohm  i_specify=off  i_priority=None  i=0 A  i_nominal_specify=off  i_nominal_unit=A  i_nominal_value=1  v_specify=off  v_priority=None  v=0 V  v_nominal_specify=off  v_nominal_unit=V  v_nominal_value=1
  Variable Resistor2 : fl_lib/Electrical/Electrical Elements/Variable Resistor  Rmin=5 Ohm  i_specify=off  i_priority=None  i=0 A  i_nominal_specify=off  i_nominal_unit=A  i_nominal_value=1  v_specify=off  v_priority=None  v=0 V  v_nominal_specify=off  v_nominal_unit=V  v_nominal_value=1
  Voltage Sensor{1..3,5,7..9} (7 alike) : fl_lib/Electrical/Electrical Sensors/Voltage Sensor
  P_PS1 : Outport
  P_WT1 : Outport  Port=2
  P_SP1 : Outport  Port=3
  P_FC1 : Outport  Port=4
  P_EL1 : Outport  Port=5
  Current : Outport  Port=6
  wires:
  PS_PWM/1 -> Saturation4/1
  WT_PWM/1 -> Saturation/1
  Divide/1 -> Simulink-PS Converter3/1, Scope8/1
  PS-Simulink Converter11/1 -> Saturation6/1
  Product11/1 -> P_EL1/1, Scope/1
  FC_PWM/1 -> Saturation3/1
  EL_PWM/1 -> Saturation2/1
  Product9/1 -> P_SP1/1, Scope3/1
  Constant5/1 -> Divide/2
  PS-Simulink Converter18/1 -> Scope6/1
  PS-Simulink Converter10/1 -> Saturation9/1
  V_WT/1 -> Simulink-PS Converter/1
  Product8/1 -> P_WT1/1, Scope2/1
  Product10/1 -> Scope4/1, P_FC1/1
  V_FC/1 -> Simulink-PS Converter1/1
  Product7/1 -> P_PS1/1, Scope1/1
  LED_PWM/1 -> Saturation1/1
  PS-Simulink Converter12/1 -> Product11/2
  PS-Simulink Converter19/1 -> Scope22/1, Saturation8/1
  PS-Simulink Converter14/1 -> Saturation5/1
  PS-Simulink Converter15/1 -> Scope7/1
  Constant3/1 -> Simulink-PS Converter4/1
  Saturation1/1 -> Divide/1
  Saturation2/1 -> Scope9/1, Subsystem5/1(In1)
  Saturation3/1 -> Subsystem7/1(In1), Scope26/1
  Saturation4/1 -> Scope19/1, Subsystem6/1(In1)
  Saturation/1 -> Scope10/1, Arduino/1(In1)
  I_SP/1 -> Scope11/1, Simulink-PS Converter2/1
  PS-Simulink Converter16/1 -> Scope21/1, Saturation7/1
  PS-Simulink Converter1/1 -> Product10/2, Product7/2, Product9/1, Product8/2, Scope14/1
  Saturation5/1 -> Scope15/1, Product8/1
  Saturation6/1 -> Product7/1, Scope20/1
  Saturation7/1 -> Scope12/1, Product9/2
  Saturation8/1 -> Product10/1, Scope17/1
  Saturation9/1 -> Product11/1, Scope16/1
  PS-Simulink Converter2/1 -> Scope23/1
  Constant/1 -> Simulink-PS Converter6/1
  DC-DC Booster1/1(Output) -> DC-DC Booster3/1(Input), DC-DC Booster2/1(Input), DC-DC Booster4/1(Input)
  DC-DC Booster3/1(Output) -> DC-DC Booster1/1(Input)
  DC-DC Booster2/1(Output) -> DC-DC Booster1/2(Input2)
  DC-DC Booster4/1(Output) -> DC-DC Booster1/3(Input1)
  PS-Simulink Converter3/1 -> Scope13/1
  PS-Simulink Converter4/1 -> Scope18/1
  DC-DC Booster3/2(Output1) -> Current/1
  connections:
  Simulink-PS Converter4/RConn1 -- Controlled Voltage Source/RConn1
  Diode9/RConn1 -- Voltage Sensor1/LConn1 -- Current Sensor8/RConn2 -- Current Sensor7/RConn2 -- Variable Resistor1/LConn2 -- Current Sensor6/RConn2 -- DC-DC Booster1/RConn1 -- " "/LConn1 -- Capacitor6/LConn1 -- Fuse1/LConn1
  Variable Resistor1/RConn1 -- DC-DC Booster4/RConn2 -- Voltage Sensor1/RConn2 -- DC-DC Booster1/RConn2 -- Resistor15/RConn1 -- Electrical Reference2/LConn1 -- DC-DC Booster3/RConn2 -- DC-DC Booster2/RConn2 -- IRLZ-34N MOSFET5/RConn2
  Capacitor2/RConn1 -- IRLZ-34N MOSFET2/RConn1 -- DC-DC Booster1/LConn2 -- Solver Configuration1/RConn1 -- Diode5/LConn1
  Diode5/RConn1 -- Resistor1/LConn1 -- Current Sensor5/RConn2
  Resistor15/LConn1 -- IRLZ-34N MOSFET5/LConn1 -- Subsystem5/RConn1
  Capacitor7/LConn1 -- DC-DC Booster4/LConn1 -- Resistor13/RConn1
  Voltage Sensor7/RConn2 -- Current Sensor9/RConn2 -- IRLZ-34N MOSFET5/RConn1 -- Electrolyzer1/RConn1
  Arduino/RConn1 -- Voltage Sensor3/LConn1 -- IRLZ-34N MOSFET3/LConn1 -- Resistor11/LConn1
  Subsystem6/RConn1 -- IRLZ-34N MOSFET2/LConn1 -- Resistor10/LConn1
  Voltage Sensor7/LConn1 -- Electrolyzer1/LConn1 -- Fuse1/RConn1
  Current Sensor9/LConn1 -- Solver Configuration3/RConn1 -- " "/RConn1 -- Diode9/LConn1 -- Capacitor6/RConn1
  DC-DC Booster2/LConn1 -- Current Sensor1/RConn2
  Capacitor7/RConn1 -- Diode8/LConn1 -- DC-DC Booster4/LConn2 -- ./RConn1
  Resistor14/LConn1 -- ./LConn1 -- Subsystem7/RConn1
  IRLZ-34N MOSFET3/RConn1 -- Voltage Sensor2/LConn1 -- DC-DC Booster3/LConn2 -- Capacitor1/RConn1
  Diode8/RConn1 -- Controlled Voltage Source2/LConn1 -- Voltage Sensor9/LConn1 -- Resistor13/LConn1
  Simulink-PS Converter3/RConn1 -- Variable Resistor1/LConn1
  PS-Simulink Converter11/LConn1 -- Current Sensor5/RConn1
  Simulink-PS Converter1/RConn1 -- Controlled Voltage Source2/RConn1
  Simulink-PS Converter/RConn1 -- Controlled Voltage Source1/RConn1
  PS-Simulink Converter18/LConn1 -- Voltage Sensor9/RConn1
  Current Sensor6/RConn1 -- PS-Simulink Converter14/LConn1
  PS-Simulink Converter15/LConn1 -- Voltage Sensor8/RConn1
  Current Sensor7/RConn1 -- PS-Simulink Converter16/LConn1
  PS-Simulink Converter19/LConn1 -- Current Sensor8/RConn1
  Controlled Voltage Source/LConn1 -- Current Sensor5/LConn1
  PS-Simulink Converter12/LConn1 -- Voltage Sensor7/RConn1
  Simulink-PS Converter2/RConn1 -- Controlled Current Source/RConn1
  PS-Simulink Converter10/LConn1 -- Current Sensor9/RConn1
  PS-Simulink Converter1/LConn1 -- Voltage Sensor1/RConn1
  Current Sensor6/LConn1 -- DC-DC Booster3/RConn1
  DC-DC Booster4/RConn1 -- Current Sensor8/LConn1
  Current Sensor7/LConn1 -- DC-DC Booster2/RConn1
  Current Sensor1/RConn1 -- PS-Simulink Converter2/LConn1
  Controlled Current Source/RConn2 -- Electrical Reference1/LConn1 -- DC-DC Booster2/LConn2
  Variable Resistor2/RConn1 -- Voltage Sensor5/RConn2 -- Current Sensor1/LConn1
  Controlled Current Source/LConn1 -- Solver Configuration2/RConn1 -- Voltage Sensor5/LConn1 -- Variable Resistor2/LConn2
  Simulink-PS Converter6/RConn1 -- Variable Resistor2/LConn1
  Resistor11/RConn1 -- Electrical Reference/LConn1 -- Voltage Sensor8/RConn2 -- Controlled Voltage Source1/RConn2 -- Voltage Sensor3/RConn2 -- Arduino/RConn2 -- Voltage Sensor2/RConn2 -- IRLZ-34N MOSFET3/RConn2
  DC-DC Booster3/LConn1 -- Resistor2/RConn1 -- Capacitor1/LConn1
  IRLZ-34N MOSFET2/RConn2 -- Subsystem6/RConn2 -- Controlled Voltage Source/RConn2 -- Electrical Reference4/LConn1 -- Resistor10/RConn1
  Controlled Voltage Source2/RConn2 -- Voltage Sensor9/RConn2 -- Electrical Reference3/LConn1 -- Solver Configuration4/RConn1 -- ./RConn2 -- Subsystem7/RConn2 -- Resistor14/RConn1
  Capacitor2/LConn1 -- DC-DC Booster1/LConn1 -- Resistor1/RConn1
  Voltage Sensor2/RConn1 -- PS-Simulink Converter3/LConn1
  Voltage Sensor3/RConn1 -- PS-Simulink Converter4/LConn1
  Resistor2/LConn1 -- Controlled Voltage Source1/LConn1 -- Solver Configuration/RConn1 -- Voltage Sensor8/LConn1

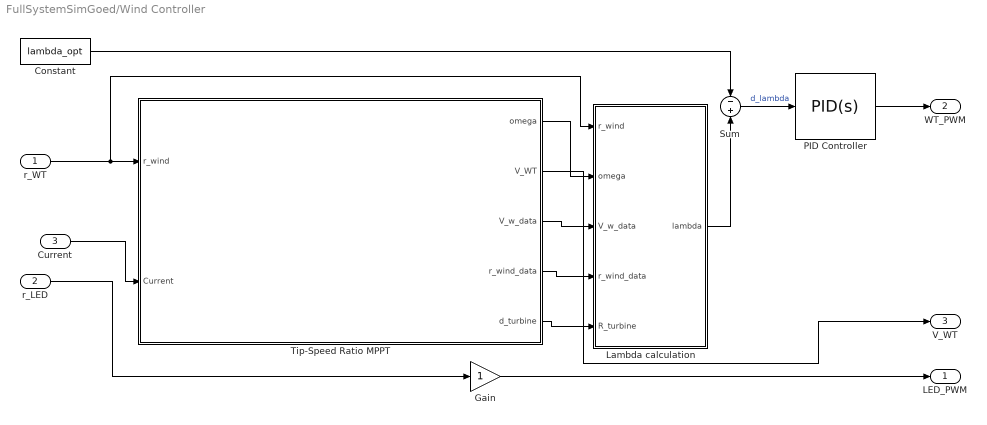
== system FullSystemSimGoed/Wind Controller ==
  r_WT : Inport
  r_LED : Inport  Port=2
  Current : Inport  Port=3
  Constant : Constant  Value=lambda_opt
  Gain : Gain
  Lambda calculation : Subsystem
  PID Controller : simulink/Continuous/PID Controller  Controller=PID  Form=Parallel  TimeDomain=Continuous-time  UseExternalTs=off  SampleTime=-1  IntegratorMethod=Forward Euler  FilterMethod=Forward Euler  ControllerParametersSource=internal  P=1  I=1  D=0  UseFilter=on  N=100  TunerSelectOption=Transfer Function Based (PID Tuner App)  InitialConditionSource=internal  InitialConditionForIntegrator=0  InitialConditionForFilter=0  DifferentiatorICPrevScaledInput=0  ExternalReset=none  TrackingMode=off  Kt=1  LimitOutput=off  UpperSaturationLimit=inf  LowerSaturationLimit=-inf  LinearizeAsGain=on  AntiWindupMode=none  Kb=1  POutMin=[]  POutMax=[]  IOutMin=[]  IOutMax=[]  DOutMin=[]  DOutMax=[]  NOutMin=[]  NOutMax=[]  SumOutMin=[]  SumOutMax=[]  SaturationOutMin=[]  SaturationOutMax=[]  PParamMin=[]  PParamMax=[]  IParamMin=[]  IParamMax=[]  DParamMin=[]  DParamMax=[]  NParamMin=[]  NParamMax=[]  KbParamMin=[]  KbParamMax=[]  KtParamMin=[]  KtParamMax=[]  KbOutMin=[]  KbOutMax=[]  KtOutMin=[]  KtOutMax=[]  IntegratorOutMin=[]  IntegratorOutMax=[]  FilterOutMin=[]  FilterOutMax=[]  SumI1OutMin=[]  SumI1OutMax=[]  SumI2OutMin=[]  SumI2OutMax=[]  SumI3OutMin=[]  SumI3OutMax=[]  SumI4OutMin=[]  SumI4OutMax=[]  SumDOutMin=[]  SumDOutMax=[]  DifferentiatorOutMin=[]  DifferentiatorOutMax=[]  FilterDiffOutCoefMin=[]  FilterDiffOutCoefMax=[]  ReciprocalOutMin=[]  ReciprocalOutMax=[]  SumDenOutMin=[]  SumDenOutMax=[]  SumNumOutMin=[]  SumNumOutMax=[]  DivideOutMin=[]  DivideOutMax=[]  UdiffTsProdOutMin=[]  UdiffTsProdOutMax=[]  NTsProdOutMin=[]  NTsProdOutMax=[]  UintegralTsProdOutMin=[]  UintegralTsProdOutMax=[]  UngainTsProdOutMin=[]  UngainTsProdOutMax=[]  IntegratorContinuousStateAttributes=''  IntegratorStateMustResolveToSignalObject=off  IntegratorRTWStateStorageClass=Auto  FilterContinuousStateAttributes=''  FilterStateMustResolveToSignalObject=off  FilterRTWStateStorageClass=Auto  ParallelPVariant=InternalParameters  IdealPVariant=Disabled  IVariant=InternalParameters  DVariant=InternalParameters  IntegratorVariant=Continuous  SatVariant=Disabled  AWVariant=Passthrough  PCopyVariant=Disabled  TRVariant=Disabled  FdbkBlocksVariant=Forward  IdealPFdbkVariant=Disabled  SatFdbkVariant=Disabled  DerivativeFilterVariant=ContFilter  NVariant=InternalParameters  NCopyVariant=Disabled  FilterICVariant=InternalICsFilter  IntegratorICVariant=InternalICs  ExternalResetVariant=Disabled  TRSumVariant=Passthrough  SumFdbkVariant=Disabled  SumVariant=Sum_PID  TsampFilterVariant=InternalTs  TsampNgainVariant=Passthrough  TsampIntegralVariant=Passthrough
  Sum : Sum  Inputs=-+
  Tip-Speed Ratio MPPT : Subsystem
  LED_PWM : Outport
  WT_PWM : Outport  Port=2
  V_WT : Outport  Port=3
  wires:
  Sum/1 -> PID Controller/1  "d_lambda"
  Tip-Speed Ratio MPPT/5(d_turbine) -> Lambda calculation/5(R_turbine)
  r_LED/1 -> Gain/1
  Tip-Speed Ratio MPPT/3(V_w_data) -> Lambda calculation/3(V_w_data)
  Tip-Speed Ratio MPPT/1(omega) -> Lambda calculation/2(omega)
  r_WT/1 -> Lambda calculation/1(r_wind), Tip-Speed Ratio MPPT/1(r_wind)
  Constant/1 -> Sum/1
  PID Controller/1 -> WT_PWM/1
  Gain/1 -> LED_PWM/1
  Tip-Speed Ratio MPPT/2(V_WT) -> V_WT/1
  Lambda calculation/1(lambda) -> Sum/2
  Tip-Speed Ratio MPPT/4(r_wind_data) -> Lambda calculation/4(r_wind_data)
  Current/1 -> Tip-Speed Ratio MPPT/2(Current)

== system FullSystemSimGoed/Hydrogen Controller/If Action Subsystem ==
  In1 : Inport
  Action Port : ActionPort  ActionPortLabel=else
  Abs : Abs
  Out1 : Outport
  wires:
  In1/1 -> Abs/1
  Abs/1 -> Out1/1

== system FullSystemSimGoed/Hydrogen Controller/If Action Subsystem1 ==
  In1 : Inport
  Action Port : ActionPort  ActionPortLabel=if(u1 > 0)
  Out1 : Outport
  wires:
  In1/1 -> Out1/1

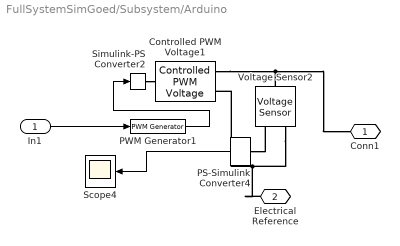
== system FullSystemSimGoed/Subsystem/Arduino ==
  In1 : Inport
  Controlled PWM Voltage1 : ee_lib/Integrated Circuits/Controlled PWM Voltage  F=10 Hz  TD=0 s  pulse_width_offset=0 s  pulse_min=0 s  Vmin=0 V  Vmax=5 V  Vm=5 V  pwm_or_av=1  event_type=1  sample_time=1e-6 s  u_min=0  u_max=1
      settings: InternalSimscapePortConfiguration="{\"Bottom\":[],\"Left\":[{\"id\":\"u\",\"label\":\"u\",\"type\":\"input\"}],\"Right\":[{\"id\":\"p2\",\"label\":\"PWM\",\"type\":\"foundation.electrical.electrical\"},{\"id\":\"n2\",\"label\":\"REF\",\"type\":\"foundation.electrical.electrical\"}],\"Top\":[]}"
  PS-Simulink Converter4 : nesl_utility/PS-Simulink Converter  PhysicalDomain=network_engine_domain  SubClassName=ps_output  LeftPortType=input  RightPortType=output  PseudoPeriodic=off  Frequencies=[]  Unit=inherit  AffineConversion=off
  PWM Generator1 : eePwmGenerator/PWM Generator  CarrCount=Up  Tper=pwm_timer  Ts=t_sample
  Scope4 : Scope
  Simulink-PS Converter2 : nesl_utility/Simulink-PS Converter  PhysicalDomain=network_engine_domain  SubClassName=ps_input  LeftPortType=input  RightPortType=output  PseudoPeriodic=off  Frequencies=[]  NoiseDistribution=none  NoiseParameters=[]  Unit=1  AffineConversion=off  FilteringAndDerivatives=provide  SimscapeFilterOrder=1  InputFilterTimeConstant=0.001  UdotUserProvided=0
  Voltage Sensor2 : fl_lib/Electrical/Electrical Sensors/Voltage Sensor
  Conn1 : PMIOPort  Side=Right
  Electrical Reference : PMIOPort  Port=2  Side=Right
  wires:
  In1/1 -> PWM Generator1/1
  PWM Generator1/1 -> Simulink-PS Converter2/1
  PS-Simulink Converter4/1 -> Scope4/1
  connections:
  PS-Simulink Converter4/LConn1 -- Voltage Sensor2/RConn1
  Voltage Sensor2/RConn2 -- Electrical Reference/RConn1 -- Controlled PWM Voltage1/RConn2
  Controlled PWM Voltage1/RConn1 -- Conn1/RConn1 -- Voltage Sensor2/LConn1
  Simulink-PS Converter2/RConn1 -- Controlled PWM Voltage1/LConn1

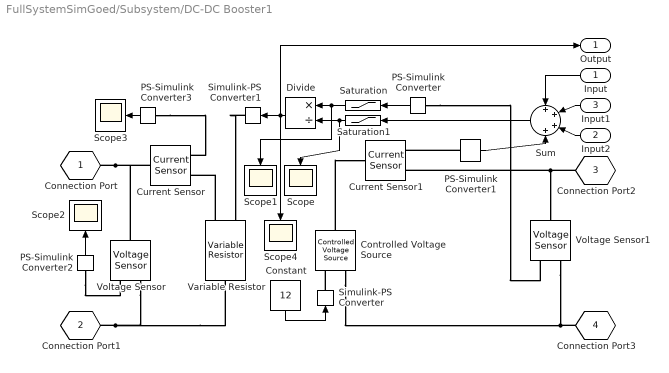
== system FullSystemSimGoed/Subsystem/DC-DC Booster1 ==
  Input : Inport
  Input2 : Inport  Port=2
  Input1 : Inport  Port=3
  Constant : Constant  Value=12
  Controlled Voltage Source : fl_lib/Electrical/Electrical Sources/Controlled Voltage Source
  Current Sensor : fl_lib/Electrical/Electrical Sensors/Current Sensor
  Current Sensor1 : fl_lib/Electrical/Electrical Sensors/Current Sensor
  Divide : Product  Inputs=*/
  PS-Simulink Converter{,1..3} (4 alike) : nesl_utility/PS-Simulink Converter  PhysicalDomain=network_engine_domain  SubClassName=ps_output  LeftPortType=input  RightPortType=output  PseudoPeriodic=off  Frequencies=[]  Unit=inherit  AffineConversion=off
  Saturation : Saturate  UpperLimit=13  LowerLimit=0
  Saturation1 : Saturate  UpperLimit=2  LowerLimit=0.01
  Scope{,1..4} (5 alike) : Scope
  Simulink-PS Converter : nesl_utility/Simulink-PS Converter  PhysicalDomain=network_engine_domain  SubClassName=ps_input  LeftPortType=input  RightPortType=output  PseudoPeriodic=off  Frequencies=[]  NoiseDistribution=none  NoiseParameters=[]  Unit=1  AffineConversion=off  FilteringAndDerivatives=provide  SimscapeFilterOrder=1  InputFilterTimeConstant=0.001  UdotUserProvided=0
  Simulink-PS Converter1 : nesl_utility/Simulink-PS Converter  PhysicalDomain=network_engine_domain  SubClassName=ps_input  LeftPortType=input  RightPortType=output  PseudoPeriodic=off  Frequencies=[]  NoiseDistribution=none  NoiseParameters=[]  Unit=1  AffineConversion=off  FilteringAndDerivatives=provide  SimscapeFilterOrder=1  InputFilterTimeConstant=0.001  UdotUserProvided=0
  Sum : Sum  Inputs=++++
  Variable Resistor : fl_lib/Electrical/Electrical Elements/Variable Resistor  Rmin=0 Ohm  i_specify=off  i_priority=None  i=0 A  i_nominal_specify=off  i_nominal_unit=A  i_nominal_value=1  v_specify=off  v_priority=None  v=0 V  v_nominal_specify=off  v_nominal_unit=V  v_nominal_value=1
  Voltage Sensor : fl_lib/Electrical/Electrical Sensors/Voltage Sensor
  Voltage Sensor1 : fl_lib/Electrical/Electrical Sensors/Voltage Sensor
  Connection Port : PMIOPort  Tag=PMCPort  Side=Left
  Connection Port1 : PMIOPort  Tag=PMCPort  Port=2  Side=Left
  Connection Port2 : PMIOPort  Tag=PMCPort  Port=3  Side=Right
  Connection Port3 : PMIOPort  Tag=PMCPort  Port=4  Side=Right
  Output : Outport
  wires:
  Constant/1 -> Simulink-PS Converter/1
  PS-Simulink Converter2/1 -> Scope2/1
  PS-Simulink Converter3/1 -> Scope3/1
  Saturation/1 -> Scope1/1, Divide/1
  PS-Simulink Converter/1 -> Saturation/1
  Saturation1/1 -> Scope/1, Divide/2
  Divide/1 -> Output/1, Scope4/1, Simulink-PS Converter1/1
  Sum/1 -> Saturation1/1
  PS-Simulink Converter1/1 -> Sum/4
  Input/1 -> Sum/1
  Input1/1 -> Sum/2
  Input2/1 -> Sum/3
  connections:
  Voltage Sensor1/RConn2 -- Controlled Voltage Source/RConn2 -- Connection Port3/RConn1
  Connection Port1/RConn1 -- Voltage Sensor/RConn2 -- Variable Resistor/RConn1
  Connection Port/RConn1 -- Current Sensor/LConn1 -- Voltage Sensor/LConn1
  Simulink-PS Converter1/RConn1 -- Variable Resistor/LConn1
  Simulink-PS Converter/RConn1 -- Controlled Voltage Source/RConn1
  PS-Simulink Converter1/LConn1 -- Current Sensor1/RConn1
  Variable Resistor/LConn2 -- Current Sensor/RConn2
  PS-Simulink Converter/LConn1 -- Voltage Sensor1/RConn1
  PS-Simulink Converter2/LConn1 -- Voltage Sensor/RConn1
  PS-Simulink Converter3/LConn1 -- Current Sensor/RConn1
  Controlled Voltage Source/LConn1 -- Current Sensor1/LConn1
  Connection Port2/RConn1 -- Current Sensor1/RConn2 -- Voltage Sensor1/LConn1

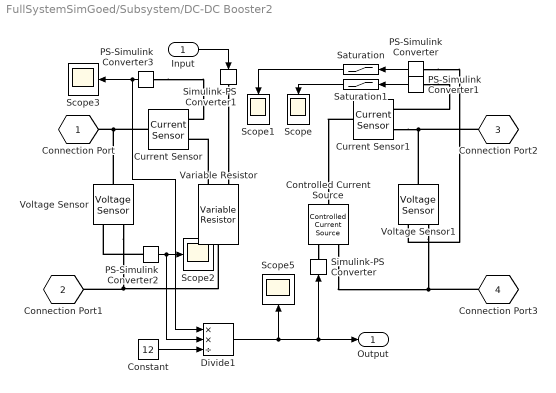
== system FullSystemSimGoed/Subsystem/DC-DC Booster2 ==
  Input : Inport
  Constant : Constant  Value=12
  Controlled Current Source : fl_lib/Electrical/Electrical Sources/Controlled Current Source
  Current Sensor : fl_lib/Electrical/Electrical Sensors/Current Sensor
  Current Sensor1 : fl_lib/Electrical/Electrical Sensors/Current Sensor
  Divide1 : Product  Inputs=**/
  PS-Simulink Converter{,1..3} (4 alike) : nesl_utility/PS-Simulink Converter  PhysicalDomain=network_engine_domain  SubClassName=ps_output  LeftPortType=input  RightPortType=output  PseudoPeriodic=off  Frequencies=[]  Unit=inherit  AffineConversion=off
  Saturation : Saturate  UpperLimit=13  LowerLimit=0
  Saturation1 : Saturate  UpperLimit=2  LowerLimit=0
  Scope{,1..3,5} (5 alike) : Scope
  Simulink-PS Converter : nesl_utility/Simulink-PS Converter  PhysicalDomain=network_engine_domain  SubClassName=ps_input  LeftPortType=input  RightPortType=output  PseudoPeriodic=off  Frequencies=[]  NoiseDistribution=none  NoiseParameters=[]  Unit=1  AffineConversion=off  FilteringAndDerivatives=filter  SimscapeFilterOrder=1  InputFilterTimeConstant=0.001  UdotUserProvided=0
  Simulink-PS Converter1 : nesl_utility/Simulink-PS Converter  PhysicalDomain=network_engine_domain  SubClassName=ps_input  LeftPortType=input  RightPortType=output  PseudoPeriodic=off  Frequencies=[]  NoiseDistribution=none  NoiseParameters=[]  Unit=1  AffineConversion=off  FilteringAndDerivatives=provide  SimscapeFilterOrder=1  InputFilterTimeConstant=0.001  UdotUserProvided=0
  Variable Resistor : fl_lib/Electrical/Electrical Elements/Variable Resistor  Rmin=0 Ohm  i_specify=off  i_priority=None  i=0 A  i_nominal_specify=off  i_nominal_unit=A  i_nominal_value=1  v_specify=off  v_priority=None  v=0 V  v_nominal_specify=off  v_nominal_unit=V  v_nominal_value=1
  Voltage Sensor : fl_lib/Electrical/Electrical Sensors/Voltage Sensor
  Voltage Sensor1 : fl_lib/Electrical/Electrical Sensors/Voltage Sensor
  Connection Port : PMIOPort  Tag=PMCPort  Side=Left
  Connection Port1 : PMIOPort  Tag=PMCPort  Port=2  Side=Left
  Connection Port2 : PMIOPort  Tag=PMCPort  Port=3  Side=Right
  Connection Port3 : PMIOPort  Tag=PMCPort  Port=4  Side=Right
  Output : Outport
  wires:
  Saturation/1 -> Scope1/1
  PS-Simulink Converter/1 -> Saturation/1
  PS-Simulink Converter1/1 -> Saturation1/1
  Saturation1/1 -> Scope/1
  Constant/1 -> Divide1/3
  PS-Simulink Converter2/1 -> Divide1/2, Scope2/1
  PS-Simulink Converter3/1 -> Scope3/1, Divide1/1
  Divide1/1 -> Output/1, Simulink-PS Converter/1, Scope5/1
  Input/1 -> Simulink-PS Converter1/1
  connections:
  Connection Port3/RConn1 -- Voltage Sensor1/RConn2 -- Controlled Current Source/RConn2
  Current Sensor1/RConn2 -- Connection Port2/RConn1 -- Voltage Sensor1/LConn1
  Voltage Sensor/RConn2 -- Variable Resistor/RConn1 -- Connection Port1/RConn1
  Current Sensor/LConn1 -- Voltage Sensor/LConn1 -- Connection Port/RConn1
  Simulink-PS Converter1/RConn1 -- Variable Resistor/LConn1
  Controlled Current Source/RConn1 -- Simulink-PS Converter/RConn1
  PS-Simulink Converter1/LConn1 -- Current Sensor1/RConn1
  Variable Resistor/LConn2 -- Current Sensor/RConn2
  PS-Simulink Converter/LConn1 -- Voltage Sensor1/RConn1
  PS-Simulink Converter2/LConn1 -- Voltage Sensor/RConn1
  PS-Simulink Converter3/LConn1 -- Current Sensor/RConn1
  Current Sensor1/LConn1 -- Controlled Current Source/LConn1
